simulink model "twistlocks_logic_test"  (R2019a)
settings: Solver=VariableStepAuto  StartTime=0.0  StopTime=60  RelTol=1e-3
undefined symbols (not defined in the file): H_c, M_c_max, M_c_min, M_s, overload
settings Model: Creator=Facundo  LastModifiedBy=Facundo

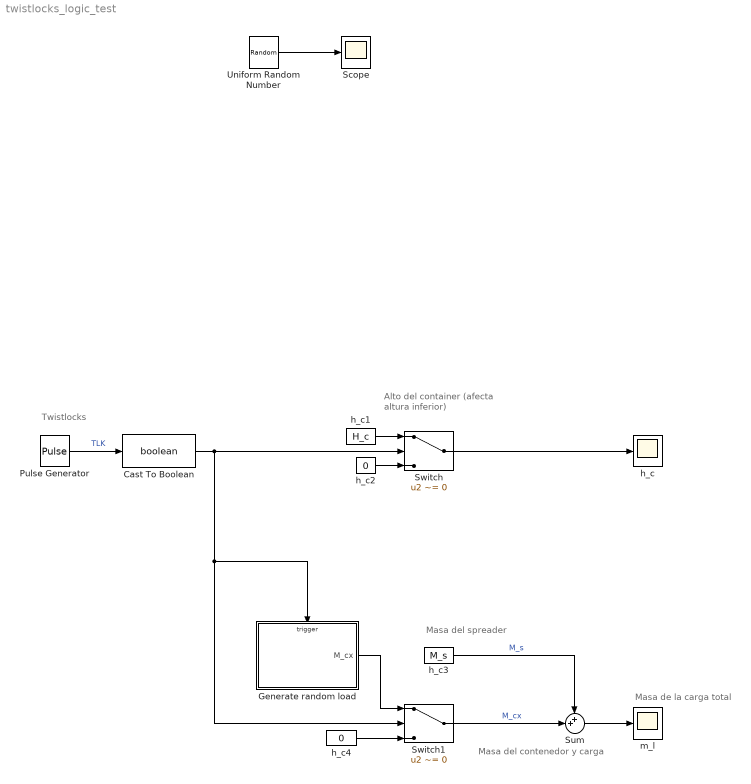
== system twistlocks_logic_test ==
  note: Masa del spreader
  note: Masa de la carga total
  note: Masa del contenedor
      | y carga
  note: Alto del container
      | (afecta altura inferior)
  note: Twistlocks
  Cast To Boolean : DataTypeConversion  OutDataTypeStr=boolean
  "Generate random load " : Subsystem  TreatAsAtomicUnit=on
  Pulse Generator : DiscretePulseGenerator  PulseType=Time based  Period=5  PulseWidth=25  PhaseDelay=2
  Scope : Scope
  Sum : Sum  Inputs=++|
  Switch : Switch  Criteria=u2 ~= 0
  Switch1 : Switch  Criteria=u2 ~= 0
  Uniform Random Number : UniformRandomNumber  SampleTime=0.1
  h_c : Scope
  h_c1 : Constant  Value=H_c
  h_c2 : Constant  Value=0
  h_c3 : Constant  Value=M_s
  h_c4 : Constant  Value=0
  m_l : Scope
  wires:
  Uniform Random Number/1 -> Scope/1
  h_c3/1 -> Sum/1  "M_s"
  "Generate random load "/1(M_cx) -> Switch1/1
  Switch1/1 -> Sum/2  "M_cx"
  Switch/1 -> h_c/1
  h_c2/1 -> Switch/3
  Sum/1 -> m_l/1
  h_c1/1 -> Switch/1
  Pulse Generator/1 -> Cast To Boolean/1  "TLK"
  h_c4/1 -> Switch1/3
  Cast To Boolean/1 -> "Generate random load "/Trigger, Switch1/2, Switch/2

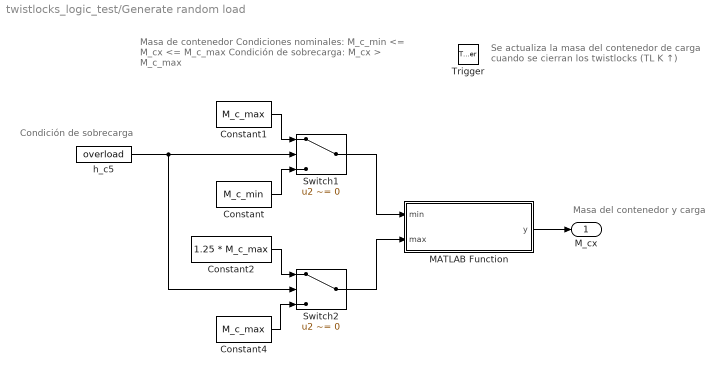
== system twistlocks_logic_test/Generate random load  ==
  note: Masa de contenedor
      | Condiciones nominales: M_c_min <= M_cx <= M_c_max
      | Condición de sobrecarga: M_cx > M_c_max
  note: Condición de sobrecarga
  note: Masa del contenedor y carga
  note: Se actualiza la masa del contenedor de carga
      | cuando se cierran los twistlocks (TL K ↑)
  Trigger : TriggerPort  VariantControl=Variant  PortDimensions=1
  Constant : Constant  Value=M_c_min
  Constant1 : Constant  Value=M_c_max
  Constant2 : Constant  Value=1.25 * M_c_max
  Constant4 : Constant  Value=M_c_max
  MATLAB Function : MATLAB Function  TreatAsAtomicUnit=on
  Switch1 : Switch  Criteria=u2 ~= 0
  Switch2 : Switch  Criteria=u2 ~= 0
  h_c5 : Constant  Value=overload
  M_cx : Outport  OutDataTypeStr=double  PortDimensions=1  InitialOutput=0
  wires:
  MATLAB Function/1(y) -> M_cx/1
  Constant/1 -> Switch1/3
  Constant1/1 -> Switch1/1
  Constant2/1 -> Switch2/1
  Constant4/1 -> Switch2/3
  h_c5/1 -> Switch1/2, Switch2/2
  Switch1/1 -> MATLAB Function/1(min)
  Switch2/1 -> MATLAB Function/2(max)

== matlab function twistlocks_logic_test/Generate random load /MATLAB Function ==
  data: y output; min input; max input
function y = update_random(min, max)
    persistent r;
    if isempty(r)
        rng('shuffle'); % Shuffle the seed ONCE at the start
    end
    r = randi([min, max]); % Generate a new random integer on trigger
    y = r;
end
